simulink model "Problema_b"  (R2023b)
settings: Solver=VariableStepAuto  StartTime=0.0  StopTime=10.0  RelTol=1e-3
settings Model: Creator=porti  LastModifiedBy=porti

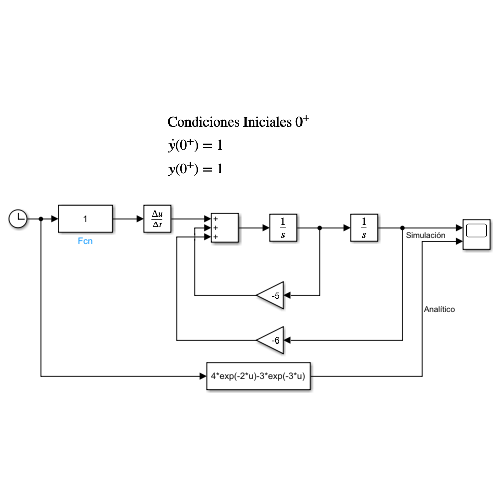
[thumbnail: Simulink's stored preview of the top-level diagram]
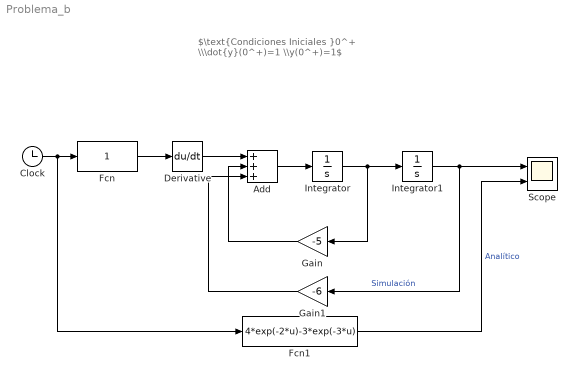
== system Problema_b ==
  note: $\text{Condiciones Iniciales }0^+ \\\dot{y}(0^+)=1 \\y(0^+)=1$
  Add : Sum  Inputs=+++
  Clock : Clock
  Derivative : Derivative
  Fcn : Fcn  Expr=1
  Fcn1 : Fcn  Expr=4*exp(-2*u)-3*exp(-3*u)
  Gain : Gain  Gain=-5
  Gain1 : Gain  Gain=-6
  Integrator : Integrator  InitialCondition=1
  Integrator1 : Integrator  InitialCondition=1
  Scope : Scope  NumInputPorts=2
  wires:
  Clock/1 -> Fcn1/1, Fcn/1
  Derivative/1 -> Add/1
  Fcn/1 -> Derivative/1
  Add/1 -> Integrator/1
  Integrator/1 -> Integrator1/1, Gain/1
  Gain/1 -> Add/2
  Integrator1/1 -> Gain1/1, Scope/1  "Simulación"
  Gain1/1 -> Add/3
  Fcn1/1 -> Scope/2  "Analítico"
